simulink model "fengliji"  (Simulink 8.1)
settings: Solver=ode45  StartTime=0.0  StopTime=10.0  RelTol=1e-3
libraries: simulink x1
settings Model: Creator=apple  LastModifiedBy=apple
settings OptimizationCC: ExpressionDepthLimit=128  InitFltsAndDblsToZero=on
settings DebuggingCC: SaveWithParameterizedLinksMsg=none  SignalResolutionControl=TryResolveAllWithWarning  MultiTaskDSMMsg=warning  MultiTaskCondExecSysMsg=none  StrictBusMsg=None
settings RTWCC: IncludeERTFirstTime=on
settings GRTTargetCC: TargetFcnLib=ansi_tfl_tmw.mat

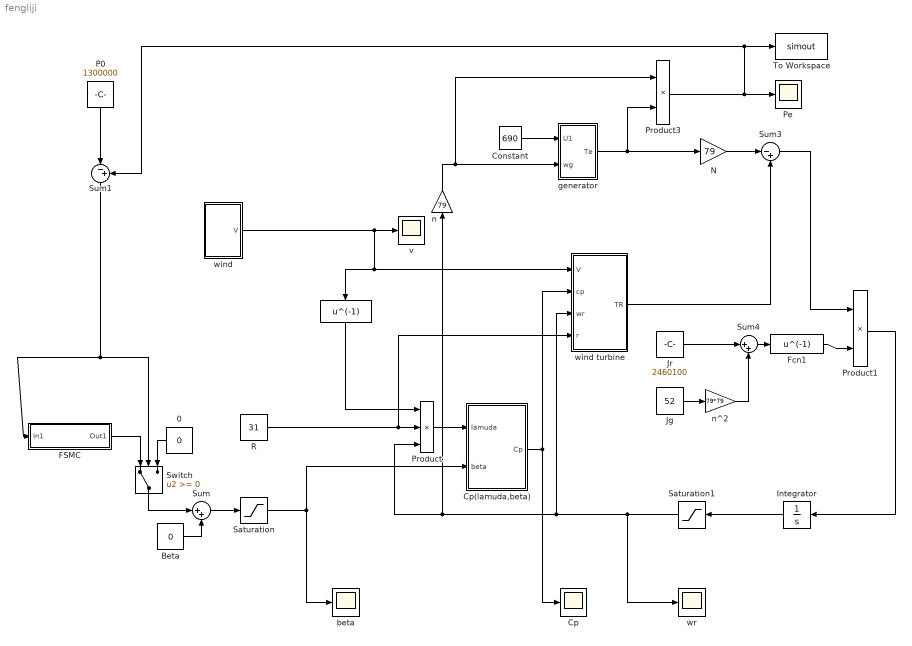
== system fengliji ==
  " " : Fcn  Expr=u^(-1)
  " Fcn1" : Fcn  Expr=u^(-1)
  0 : Constant  Value=0
  Beta : Constant  Value=0
  Constant : Constant  Value=690
  "Cp " : Scope
  Cp(lamuda,beta) : Subsystem
  FSMC : Subsystem
  Integrator : Integrator
  "Jg " : Constant  Value=52
  Jr : Constant  Value=2460100
  N : Gain  Gain=79
  P0 : Constant  Value=1300000
  Pe : Scope
      settings: SaveName=ScopeData4
  Product : Product  Inputs=3  RndMeth=Zero
  Product1 : Product  RndMeth=Zero
  Product3 : Product  RndMeth=Zero
  R : Constant  Value=31
  Saturation : Saturate
  Saturation1 : Saturate
  Sum : Sum  Inputs=|++
  Sum1 : Sum  Inputs=|-+
  Sum3 : Sum  Inputs=|-+
  Sum4 : Sum  Inputs=|++
  Switch : Switch
  To Workspace : ToWorkspace  VariableName=simout  SampleTime=-1  SaveFormat=Structure
  beta : Scope
  generator : Subsystem
  n : Gain  Gain=79
  n^2 : Gain  Gain=79*79
  v : Scope
      settings: SaveName=ScopeData2
  wind : Subsystem
  wind turbine : Subsystem
  wr : Scope
      settings: SaveName=ScopeData3
  wires:
  Cp(lamuda,beta)/1(Cp) -> "Cp "/1, wind turbine/2(cp)
  Saturation/1 -> beta/1, Cp(lamuda,beta)/2(beta)
  R/1 -> Product/2, wind turbine/4("r ")
  Product/1 -> Cp(lamuda,beta)/1(lamuda)
  Switch/1 -> Sum/1
  FSMC/1(Out1) -> Switch/1
  0/1 -> Switch/3
  Sum1/1 -> Switch/2, FSMC/1(In1)
  P0/1 -> Sum1/1
  Beta/1 -> Sum/2
  Sum/1 -> Saturation/1
  " "/1 -> Product/1
  "Jg "/1 -> n^2/1
  n^2/1 -> Sum4/2
  Jr/1 -> Sum4/1
  Sum4/1 -> " Fcn1"/1
  " Fcn1"/1 -> Product1/2
  Product1/1 -> Integrator/1
  Integrator/1 -> Saturation1/1
  Saturation1/1 -> wind turbine/3(wr), Product/3, n/1, wr/1
  generator/1(Te) -> N/1, Product3/2
  N/1 -> Sum3/1
  wind turbine/1(TR) -> Sum3/2
  Sum3/1 -> Product1/1
  n/1 -> Product3/1, generator/2(wg)
  Product3/1 -> Pe/1, To Workspace/1, Sum1/2
  Constant/1 -> generator/1(U1)
  wind/1(V) -> v/1, wind turbine/1(V), " "/1

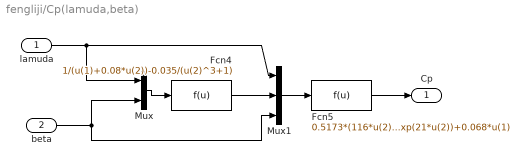
== system fengliji/Cp(lamuda,beta) ==
  lamuda : Inport
  beta : Inport  Port=2
  Fcn4 : Fcn  Expr=1/(u(1)+0.08*u(2))-0.035/(u(2)^3+1)
  Fcn5 : Fcn  Expr=0.5173*(116*u(2)-0.4*u(3)-5)*exp(21*u(2))+0.068*u(1)
  Mux : Mux  Inputs=2
  Mux1 : Mux  Inputs=3
  Cp : Outport
  wires:
  beta/1 -> Mux/2, Mux1/3
  lamuda/1 -> Mux1/1, Mux/1
  Mux/1 -> Fcn4/1
  Fcn4/1 -> Mux1/2
  Mux1/1 -> Fcn5/1
  Fcn5/1 -> Cp/1

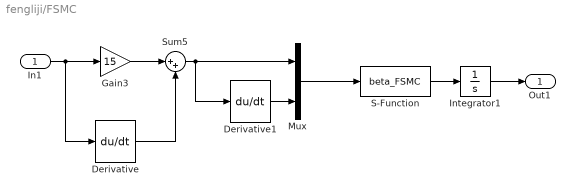
== system fengliji/FSMC ==
  In1 : Inport
  Derivative : Derivative
  Derivative1 : Derivative
  Gain3 : Gain  Gain=15
  Integrator1 : Integrator
  Mux : Mux  Inputs=2
  S-Function : S-Function  FunctionName=beta_FSMC  EnableBusSupport=off
  Sum5 : Sum  Inputs=|++
  Out1 : Outport
  wires:
  Gain3/1 -> Sum5/1
  In1/1 -> Derivative/1, Gain3/1
  Derivative/1 -> Sum5/2
  Sum5/1 -> Mux/1, Derivative1/1
  Derivative1/1 -> Mux/2
  Mux/1 -> S-Function/1
  S-Function/1 -> Integrator1/1
  Integrator1/1 -> Out1/1

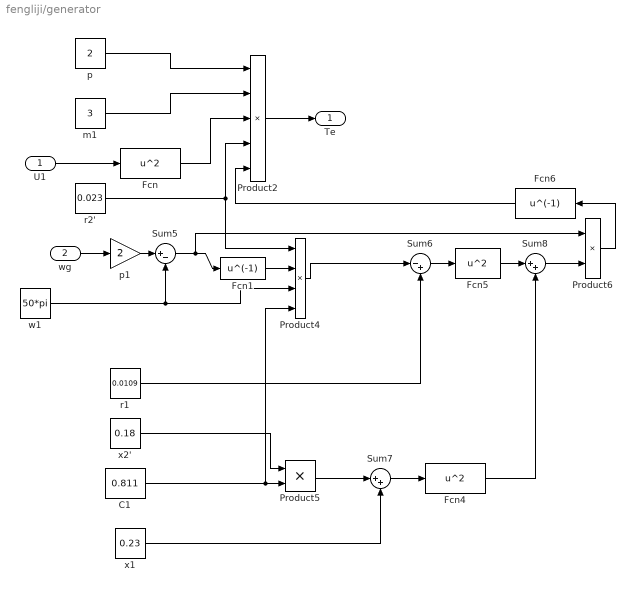
== system fengliji/generator ==
  U1 : Inport
  wg : Inport  Port=2
  C1 : Constant  Value=0.811
  Fcn : Fcn  Expr=u^2
  Fcn1 : Fcn  Expr=u^(-1)
  Fcn4 : Fcn  Expr=u^2
  Fcn5 : Fcn  Expr=u^2
  Fcn6 : Fcn  Expr=u^(-1)
  Product2 : Product  Inputs=5  RndMeth=Zero
  Product4 : Product  Inputs=4  RndMeth=Zero
  Product5 : Product  RndMeth=Zero
  Product6 : Product  RndMeth=Zero
  Sum5 : Sum  Inputs=|+-
  Sum6 : Sum  Inputs=|-+
  Sum7 : Sum  Inputs=|++
  Sum8 : Sum  Inputs=|++
  m1 : Constant  Value=3
  p : Constant  Value=2
  p1 : Gain  Gain=2
  r1 : Constant  Value=0.0109
  r2' : Constant  Value=0.023
  w1 : Constant  Value=50*pi
  x1 : Constant  Value=0.23
  x2' : Constant  Value=0.18
  Te : Outport
  wires:
  U1/1 -> Fcn/1
  p/1 -> Product2/1
  m1/1 -> Product2/2
  Fcn/1 -> Product2/3
  r2'/1 -> Product2/4, Product4/1
  Product2/1 -> Te/1
  wg/1 -> p1/1
  p1/1 -> Sum5/1
  w1/1 -> Product4/3, Sum5/2
  Sum5/1 -> Fcn1/1, Product6/1
  Fcn1/1 -> Product4/2
  C1/1 -> Product4/4, Product5/2
  x2'/1 -> Product5/1
  Product5/1 -> Sum7/1
  x1/1 -> Sum7/2
  Sum7/1 -> Fcn4/1
  Product4/1 -> Sum6/1
  r1/1 -> Sum6/2
  Sum6/1 -> Fcn5/1
  Fcn5/1 -> Sum8/1
  Fcn4/1 -> Sum8/2
  Sum8/1 -> Product6/2
  Product6/1 -> Fcn6/1
  Fcn6/1 -> Product2/5

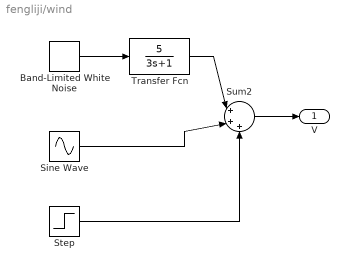
== system fengliji/wind ==
  Band-Limited White Noise : simulink/Sources/Band-Limited White Noise  Cov=[0.1]  Ts=0.1  seed=[23341]
  Sine Wave : Sin  Amplitude=3  Frequency=0.2  SampleTime=0
  Step : Step  Time=40  Before=8  After=13  SampleTime=0
  Sum2 : Sum  Inputs=|+++
  Transfer Fcn : TransferFcn  Numerator=[5]  Denominator=[3 1]
  V : Outport
  wires:
  Sine Wave/1 -> Sum2/2
  Band-Limited White Noise/1 -> Transfer Fcn/1
  Step/1 -> Sum2/3
  Sum2/1 -> V/1
  Transfer Fcn/1 -> Sum2/1

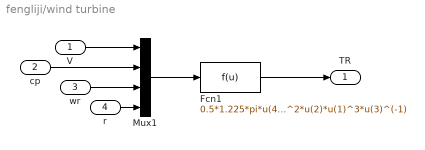
== system fengliji/wind turbine ==
  V : Inport
  cp : Inport  Port=2
  wr : Inport  Port=3
  "r " : Inport  Port=4
  Fcn1 : Fcn  Expr=0.5*1.225*pi*u(4)^2*u(2)*u(1)^3*u(3)^(-1)
  Mux1 : Mux
  TR : Outport
  wires:
  cp/1 -> Mux1/2
  V/1 -> Mux1/1
  wr/1 -> Mux1/3
  Mux1/1 -> Fcn1/1
  Fcn1/1 -> TR/1
  "r "/1 -> Mux1/4
